simulink library "HDL_ieee_8021513"  (R2024a)
settings: Solver=FixedStepDiscrete  StartTime=0.0  StopTime=10.0  RelTol=1e-3
undefined symbols (not defined in the file): Add, axiWidth, CONST, fs, peakDetectorThreshold, peakDetectorWindow, QAM, Shift
libraries: hdlsllib x199, $bdroot x91, whdlutilities x34, whdledac x9, simulink x8, whdlmod x6, dspsigops x5, dsphdlfiltering2 x4, embreciprocals x3, dsphdlsigops2 x2, commhdlcrc x2, dspstat3 x2
(part 4 of 6)

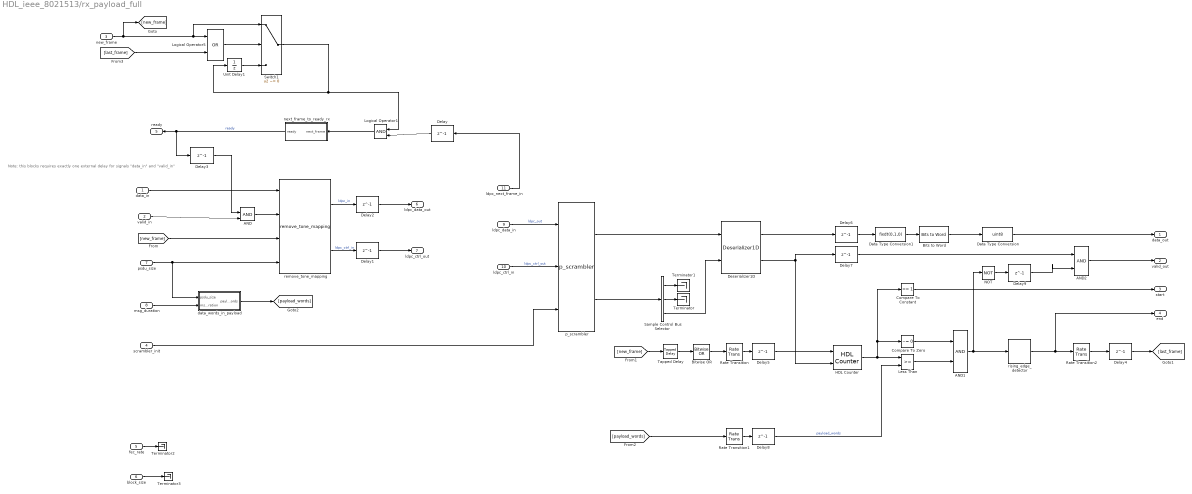
== system HDL_ieee_8021513/rx_payload_full ==
  note: Note: this blocks requires exactly one external delay for signals "data_in" and "valid_in"
  data_in : Inport
  valid_in : Inport  Port=2
  new_frame : Inport  Port=3
  scrambler_init : Inport  Port=4
  fec_rate : Inport  Port=5
  block_size : Inport  Port=6
  psdu_size : Inport  Port=7
  msg_duration : Inport  Port=8
  ldpc_data_in : Inport  Port=9
  ldpc_ctrl_in : Inport  Port=10
  ldpc_next_frame_in : Inport  Port=11
  AND : Logic  IconShape=distinctive  AllPortsSameDT=off  OutDataTypeStr=boolean
  AND1 : Logic  IconShape=distinctive  AllPortsSameDT=off  OutDataTypeStr=boolean
  AND2 : Logic  IconShape=distinctive  AllPortsSameDT=off  OutDataTypeStr=boolean
  Bits to Word : hdlsllib/Logic and Bit Operations/Bits to Word
  Bitwise OR : simulink/Logic and Bit Operations/Bitwise Operator  logicop=OR  UseBitMask=off  BitMask=bin2dec('11011001')  BitMaskRealWorld=Stored Integer
      settings: LibrarySourceBlock=|
      | simulink/Quick Insert/Logic and Bit
      | Operations/Bitwise OR
  Compare To Constant : hdlsllib/Logic and Bit Operations/Compare To Constant  relop===  const=1  OutDataTypeStr=boolean
  Compare To Zero : hdlsllib/Logic and Bit Operations/Compare To Zero  relop=~=  OutDataTypeStr=boolean
  Data Type Conversion : DataTypeConversion  OutDataTypeStr=uint8  SaturateOnIntegerOverflow=off  RndMeth=Floor
  Data Type Conversion1 : DataTypeConversion  OutDataTypeStr=fixdt(0,1,0)  SaturateOnIntegerOverflow=off  RndMeth=Floor
  Delay{,1..9} (10 alike) : Delay  DelayLength=1  InitialCondition=0  UseCircularBuffer=on
  Deserializer1D : hdlsllib/HDL Operations/Deserializer1D  Ratio=8  IdleCycles=0  InitialCondition=0  startIn=off  validIn=on  validOut=on  inputDataDimensions=-1  inputSampleTime=-1  inputSignalType=auto
  HDL Counter : hdlsllib/Sources/HDL Counter  CountType=Free running  CountInit=0  CountStep=1  CountMax=25  CountFromType=Initial value  CountFrom=0  CountResetPort=on  CountLoadPort=off  CountEnbPort=on  CountDirPort=off  CountHitOutputPort=off  CountDataType=Unsigned  CountWordLen=32  CountFracLen=0  CountSampTime=1
  Less Than : RelationalOperator  OutDataTypeStr=boolean  RndMeth=Simplest  InputSameDT=off
  Logical Operator1 : Logic  IconShape=distinctive  AllPortsSameDT=off  OutDataTypeStr=boolean
  Logical Operator5 : Logic  Operator=OR  IconShape=distinctive  AllPortsSameDT=off  OutDataTypeStr=boolean
  NOT : Logic  Operator=NOT  IconShape=distinctive  AllPortsSameDT=off  OutDataTypeStr=boolean
  Rate Transition : RateTransition  OutPortSampleTimeOpt=Multiple of input port sample time  OutPortSampleTimeMultiple=8
  Rate Transition1 : RateTransition  OutPortSampleTimeOpt=Multiple of input port sample time  OutPortSampleTimeMultiple=8
  Rate Transition2 : RateTransition  OutPortSampleTimeOpt=Multiple of input port sample time  OutPortSampleTimeMultiple=1/8
  Sample Control Bus Selector : whdlutilities/Sample Control Bus Selector  OutputSignals=start,end,valid
  Switch1 : Switch  Criteria=u2 ~= 0  SaturateOnIntegerOverflow=off  InputSameDT=off
  Tapped Delay : simulink/Discrete/Tapped Delay  vinit=0.0  samptime=-1  NumDelays=8  DelayOrder=Oldest  includeCurrent=off
  Terminator{,1..3} (4 alike) : Terminator
  Unit Delay1 : UnitDelay  SampleTime=-1  HasFrameUpgradeWarning=on
  data_words_in_payload : Subsystem
  next_frame_to_ready_rx : Subsystem
  p_scrambler : $bdroot/p_scrambler  SystemSampleTime=-1  VariantActivationTime=update diagram  AllowFlexibleInterface=on  Latency=0  AutoFrameSizeCalculation=off
      settings: LibrarySourceBlock=|
      | hdlsllib/Ports &
      | Subsystems/Subsystem
  remove_tone_mapping : $bdroot/remove_tone_mapping  SystemSampleTime=-1  VariantActivationTime=update diagram  AllowFlexibleInterface=on  Latency=0  AutoFrameSizeCalculation=off
  rising_edge_detector : $bdroot/rising_edge_detector  SystemSampleTime=-1  VariantActivationTime=update diagram  AllowFlexibleInterface=on  Latency=0  AutoFrameSizeCalculation=off
  data_out : Outport  VectorParamsAs1DForOutWhenUnconnected=off
  valid_out : Outport  Port=2  VectorParamsAs1DForOutWhenUnconnected=off
  start : Outport  Port=3  VectorParamsAs1DForOutWhenUnconnected=off
  end : Outport  Port=4  VectorParamsAs1DForOutWhenUnconnected=off
  ready : Outport  Port=5  VectorParamsAs1DForOutWhenUnconnected=off
  ldpc_data_out : Outport  Port=6  VectorParamsAs1DForOutWhenUnconnected=off
  ldpc_ctrl_out : Outport  Port=7  VectorParamsAs1DForOutWhenUnconnected=off
  wires:
  Delay6/1 -> Data Type Conversion1/1
  Delay9/1 -> AND2/2
  NOT/1 -> Delay9/1
  AND2/1 -> valid_out/1
  Delay7/1 -> AND2/1
  Compare To Zero/1 -> AND1/1
  Less Than/1 -> AND1/2
  AND1/1 -> rising_edge_detector/1, NOT/1
  Compare To Constant/1 -> start/1
  Delay4/1 -> [last_frame]
  Rate Transition2/1 -> Delay4/1
  rising_edge_detector/1 -> Rate Transition2/1, end/1
  Delay8/1 -> Less Than/2  "payload_words"
  Rate Transition1/1 -> Delay8/1
  [payload_words] -> Rate Transition1/1
  Delay5/1 -> HDL Counter/1
  data_words_in_payload/1(payload_words) -> [payload_words]
  HDL Counter/1 -> Less Than/1, Compare To Zero/1, Compare To Constant/1
  Rate Transition/1 -> Delay5/1
  Bitwise OR/1 -> Rate Transition/1
  [new_frame] -> Tapped Delay/1
  Tapped Delay/1 -> Bitwise OR/1
  msg_duration/1 -> data_words_in_payload/2(msg_duration)
  Deserializer1D/1 -> Delay6/1
  Deserializer1D/2 -> HDL Counter/2, Delay7/1
  Bits to Word/1 -> Data Type Conversion/1
  block_size/1 -> Terminator3/1
  fec_rate/1 -> Terminator2/1
  Delay2/1 -> ldpc_data_out/1
  Delay1/1 -> ldpc_ctrl_out/1
  p_scrambler/2 -> Sample Control Bus Selector/1
  Sample Control Bus Selector/2 -> Terminator/1
  Sample Control Bus Selector/1 -> Terminator1/1
  scrambler_init/1 -> p_scrambler/3
  ldpc_ctrl_in/1 -> p_scrambler/2  "ldpc_ctrl_out"
  ldpc_data_in/1 -> p_scrambler/1  "ldpc_out"
  psdu_size/1 -> remove_tone_mapping/4, data_words_in_payload/1(psdu_size)
  remove_tone_mapping/1 -> Delay2/1  "ldpc_in"
  remove_tone_mapping/2 -> Delay1/1  "ldpc_ctrl_in"
  ldpc_next_frame_in/1 -> Delay/1
  next_frame_to_ready_rx/1(ready) -> Delay3/1, ready/1  "ready"
  data_in/1 -> remove_tone_mapping/1
  AND/1 -> remove_tone_mapping/2
  valid_in/1 -> AND/2
  Delay3/1 -> AND/1
  Logical Operator5/1 -> Switch1/2
  new_frame/1 -> [new_frame], Switch1/1, Logical Operator5/1
  Unit Delay1/1 -> Switch1/3
  Logical Operator1/1 -> next_frame_to_ready_rx/1(next_frame)
  Switch1/1 -> Logical Operator1/1, Unit Delay1/1
  Delay/1 -> Logical Operator1/2
  [last_frame] -> Logical Operator5/2
  [new_frame] -> remove_tone_mapping/3
  Sample Control Bus Selector/3 -> Deserializer1D/2
  Data Type Conversion/1 -> data_out/1
  p_scrambler/1 -> Deserializer1D/1
  Data Type Conversion1/1 -> Bits to Word/1

== system HDL_ieee_8021513/signal_ack ==
  signal_in : Inport
  free_signal : Inport  Port=2
  Logical Operator : Logic  Operator=OR  IconShape=distinctive  AllPortsSameDT=off  OutDataTypeStr=boolean
  Logical Operator3 : Logic  Operator=NOT  IconShape=distinctive  AllPortsSameDT=off  OutDataTypeStr=boolean
  State Control : StateControl  StateControl=Synchronous
  Switch : Switch  Criteria=u2 ~= 0  SaturateOnIntegerOverflow=off  InputSameDT=off
  Unit Delay : UnitDelay  SampleTime=-1  HasFrameUpgradeWarning=on
  rising_edge_detector : $bdroot/rising_edge_detector  SystemSampleTime=-1  VariantActivationTime=update diagram  AllowFlexibleInterface=on  Latency=0  AutoFrameSizeCalculation=off
  signal_out : Outport
  wires:
  Unit Delay/1 -> Switch/3
  Switch/1 -> Logical Operator3/1, Unit Delay/1
  Logical Operator/1 -> Switch/2
  free_signal/1 -> Logical Operator/1, Switch/1
  Logical Operator3/1 -> signal_out/1
  signal_in/1 -> rising_edge_detector/1
  rising_edge_detector/1 -> Logical Operator/2

== system HDL_ieee_8021513/tone_mapping ==
  data_in : Inport
  ctrl_in : Inport  Port=2
  bits_per_subcarrier : Inport  Port=3
  len_in_ofdm_symbols : Inport  Port=4
  new_frame : Inport  Port=5
  Compare To Constant : hdlsllib/Logic and Bit Operations/Compare To Constant  relop===  const=1  OutDataTypeStr=boolean
  Constant : Constant  Value=0  OutDataTypeStr=boolean  SampleTime=-1
  Data Type Conversion : DataTypeConversion  OutDataTypeStr=uint8  SaturateOnIntegerOverflow=off  RndMeth=Floor
  Delay{,1..4,6..7,10} (8 alike) : Delay  DelayLength=1  InitialCondition=0  UseCircularBuffer=on
  Delay{5,8..9,11..12} (5 alike) : Delay  InitialCondition=0  UseCircularBuffer=on
  Gain : Gain  Gain=CONST.numDataCarriers  OutDataTypeStr=fixdt(0,10,0)
  HDL Counter : hdlsllib/Sources/HDL Counter  CountType=Free running  CountInit=0  CountStep=1  CountMax=1  CountFromType=Initial value  CountFrom=0  CountResetPort=on  CountLoadPort=off  CountEnbPort=on  CountDirPort=off  CountHitOutputPort=off  CountDataType=Unsigned  CountWordLen=32  CountFracLen=0  CountSampTime=1
  Logical Operator : Logic  AllPortsSameDT=off  OutDataTypeStr=boolean
  Logical Operator1 : Logic  IconShape=distinctive  AllPortsSameDT=off  OutDataTypeStr=boolean
  Logical Operator{2,4,6..7} (4 alike) : Logic  Operator=OR  IconShape=distinctive  AllPortsSameDT=off  OutDataTypeStr=boolean
  Logical Operator3 : Logic  IconShape=distinctive  AllPortsSameDT=off  OutDataTypeStr=boolean
  Logical Operator5 : Logic  IconShape=distinctive  AllPortsSameDT=off  OutDataTypeStr=boolean
  Product1 : Product
  Relational Operator : RelationalOperator  Operator=<=  OutDataTypeStr=boolean  InputSameDT=off
  Sample Control Bus Creator : whdlutilities/Sample Control Bus Creator
  Sample Control Bus Selector : whdlutilities/Sample Control Bus Selector  OutputSignals=start,end,valid
  State Control : StateControl  StateControl=Synchronous
  Subtract : Sum  Inputs=+-
  Switch : Switch  Criteria=u2 ~= 0  SaturateOnIntegerOverflow=off  InputSameDT=off
  Switch1 : Switch  Criteria=u2 ~= 0  SaturateOnIntegerOverflow=off  InputSameDT=off
  Switch2 : Switch  Criteria=u2 ~= 0  SaturateOnIntegerOverflow=off  InputSameDT=off
  Unit Delay1 : UnitDelay  SampleTime=-1  HasFrameUpgradeWarning=on
  Unit Delay2 : UnitDelay  SampleTime=-1  HasFrameUpgradeWarning=on
  data_out : Outport
  ctrl_out : Outport  Port=2
  wires:
  Delay12/1 -> Delay9/1
  Delay11/1 -> Gain/1
  Data Type Conversion/1 -> Delay11/1
  Delay2/1 -> Logical Operator7/1
  Logical Operator1/1 -> Delay3/1
  Logical Operator7/1 -> Switch1/2
  Sample Control Bus Selector/1 -> Logical Operator1/2, Delay2/1
  Unit Delay2/1 -> Switch1/3
  Switch1/1 -> Unit Delay2/1, Logical Operator1/1  "new_frame_hold"
  Sample Control Bus Selector/2 -> Logical Operator/1
  Relational Operator/1 -> Logical Operator/2
  Logical Operator/1 -> Switch2/1, Logical Operator6/2
  new_frame/1 -> Logical Operator7/2, Switch1/1, HDL Counter/1  "new_frame"
  Switch/1 -> data_out/1
  ctrl_in/1 -> Delay7/1
  Sample Control Bus Selector/3 -> Delay10/1
  Sample Control Bus Creator/1 -> ctrl_out/1
  Logical Operator2/1 -> Sample Control Bus Creator/3
  Unit Delay1/1 -> Switch2/3
  Switch2/1 -> Delay1/1, Unit Delay1/1
  Logical Operator3/1 -> Sample Control Bus Creator/2
  Logical Operator4/1 -> HDL Counter/2  "enable"
  [hold_end] -> Logical Operator4/2
  Constant/1 -> Switch/1
  data_in/1 -> Delay6/1
  [hold_end] -> Logical Operator3/2
  HDL Counter/1 -> Subtract/2  "count"
  Delay/1 -> Switch/3
  Delay1/1 -> [hold_end], Logical Operator5/2, Logical Operator2/2  "hold_end"
  Delay10/1 -> Logical Operator4/1, Logical Operator2/1
  Delay3/1 -> Sample Control Bus Creator/1
  Logical Operator6/1 -> Switch2/2
  Logical Operator5/1 -> Logical Operator6/1
  [hold_end] -> Delay4/1
  Delay4/1 -> Switch/2
  Subtract/1 -> Relational Operator/1, Compare To Constant/1
  Compare To Constant/1 -> Logical Operator5/1, Logical Operator3/1
  bits_per_subcarrier/1 -> Data Type Conversion/1
  Delay5/1 -> [count_hit]  "count_hit"
  [count_hit] -> Subtract/1
  Delay6/1 -> Delay/1
  Delay7/1 -> Sample Control Bus Selector/1
  Gain/1 -> Delay8/1
  Delay8/1 -> Product1/1, Relational Operator/2
  len_in_ofdm_symbols/1 -> Delay12/1
  Product1/1 -> Delay5/1
  Delay9/1 -> Product1/2

== system HDL_ieee_8021513/tx_decimator ==
  note: The data out from this blocks is "valid" one sample, and invalid the next.
      | This blocks makes sure that the data is valid both cycles.
      | What happens is that the ZOH might sample the signal when is valid or invalid.
  data_in : Inport
  valid_in : Inport  Port=2
  Delay{,1..2,5..10} (9 alike) : Delay  DelayLength=1  InitialCondition=0  UseCircularBuffer=on
  Delay3 : Delay  DelayLength=CONST.txDecimatorDelay*3 +6  InitialCondition=0  UseCircularBuffer=on
  Delay4 : Delay  DelayLength=CONST.txDecimatorDelay/CONST.txM  InitialCondition=0  UseCircularBuffer=on
  Downsample : DownSample  N=CONST.txM  RateOptions=Allow multirate processing
  Downsample1 : DownSample  N=CONST.txM  RateOptions=Allow multirate processing
  FIR Decimator : dsphdlfiltering2/FIR Decimator  Numerator=CONST.txDecimatorFilter.Numerator  FilterStructure=Direct form systolic  DecimationFactor=CONST.txM  NumCycles=1  SimulateUsing=Code generation  roundingMode=Floor  overflowMode=off  CoefficientsDataTypeStr=fixdt(1,16)  OutputDataTypeStr=fixdt(1,16,12)  ResetInputPort=on  HDLGlobalReset=on
  Logical Operator : Logic  Operator=OR  IconShape=distinctive  AllPortsSameDT=off  OutDataTypeStr=boolean
  Logical Operator2 : Logic  IconShape=distinctive  AllPortsSameDT=off  OutDataTypeStr=boolean
  Logical Operator3 : Logic  IconShape=distinctive  AllPortsSameDT=off  OutDataTypeStr=boolean
  Logical Operator4 : Logic  Operator=NOT  IconShape=distinctive  AllPortsSameDT=off  OutDataTypeStr=boolean
  Switch : Switch  Criteria=u2 ~= 0  SaturateOnIntegerOverflow=off  InputSameDT=off
  Switch1 : Switch  Criteria=u2 ~= 0  SaturateOnIntegerOverflow=off  InputSameDT=off
  falling_edge_detector : $bdroot/falling_edge_detector  SystemSampleTime=-1  VariantActivationTime=update diagram  AllowFlexibleInterface=on  Latency=0  AutoFrameSizeCalculation=off
  rising_edge_detector : $bdroot/rising_edge_detector  SystemSampleTime=-1  VariantActivationTime=update diagram  AllowFlexibleInterface=on  Latency=0  AutoFrameSizeCalculation=off
  data_out : Outport
  valid_out : Outport  Port=2
  wires:
  rising_edge_detector/1 -> FIR Decimator/3
  Delay10/1 -> Delay5/1
  Delay1/1 -> Logical Operator/1, Delay3/1
  valid_in/1 -> Delay1/1, rising_edge_detector/1
  Downsample1/1 -> Delay2/1
  Delay3/1 -> Logical Operator/2
  Logical Operator/1 -> FIR Decimator/2
  data_in/1 -> Delay10/1  "data_in"
  Downsample/1 -> Delay8/1  "after_down"
  Delay5/1 -> FIR Decimator/1
  Delay6/1 -> Switch/3
  Delay7/1 -> Switch1/3
  Switch1/1 -> Downsample/1
  FIR Decimator/1 -> Switch/1, Delay6/1  "data_out"
  Switch/1 -> Downsample1/1
  FIR Decimator/2 -> Delay7/1, Switch/2, Switch1/1, Switch1/2  "valid_out"
  Delay/1 -> Logical Operator3/1
  Logical Operator4/1 -> Logical Operator3/2
  Delay9/1 -> data_out/1
  Logical Operator2/1 -> Delay/1, falling_edge_detector/1
  Delay8/1 -> Logical Operator2/1, Delay4/1
  Logical Operator3/1 -> valid_out/1
  falling_edge_detector/1 -> Logical Operator4/1
  Delay4/1 -> Logical Operator2/2
  Delay2/1 -> Delay9/1

== system HDL_ieee_8021513/valid_to_ctrl ==
  validIn : Inport
  Delay1 : Delay  DelayLength=1  InitialCondition=0  UseCircularBuffer=on
  Delay2 : Delay  DelayLength=1  InitialCondition=0  UseCircularBuffer=on
  Logical Operator : Logic  IconShape=distinctive  AllPortsSameDT=off  OutDataTypeStr=boolean
  Logical Operator1 : Logic  Operator=NOT  IconShape=distinctive  AllPortsSameDT=off  OutDataTypeStr=boolean
  Logical Operator2 : Logic  IconShape=distinctive  AllPortsSameDT=off  OutDataTypeStr=boolean
  Logical Operator3 : Logic  Operator=NOT  IconShape=distinctive  AllPortsSameDT=off  OutDataTypeStr=boolean
  Sample Control Bus Creator : whdlutilities/Sample Control Bus Creator
  State Control : StateControl  StateControl=Synchronous
  ctrlOut : Outport  VectorParamsAs1DForOutWhenUnconnected=off
  wires:
  validIn/1 -> Logical Operator3/1, Delay1/1
  Logical Operator3/1 -> Logical Operator2/2
  Delay2/1 -> Logical Operator1/1
  Logical Operator1/1 -> Logical Operator/2
  Delay1/1 -> Logical Operator/1, Sample Control Bus Creator/3, Logical Operator2/1, Delay2/1  "valid"
  Logical Operator/1 -> Sample Control Bus Creator/1  "start"
  Logical Operator2/1 -> Sample Control Bus Creator/2  "end"
  Sample Control Bus Creator/1 -> ctrlOut/1

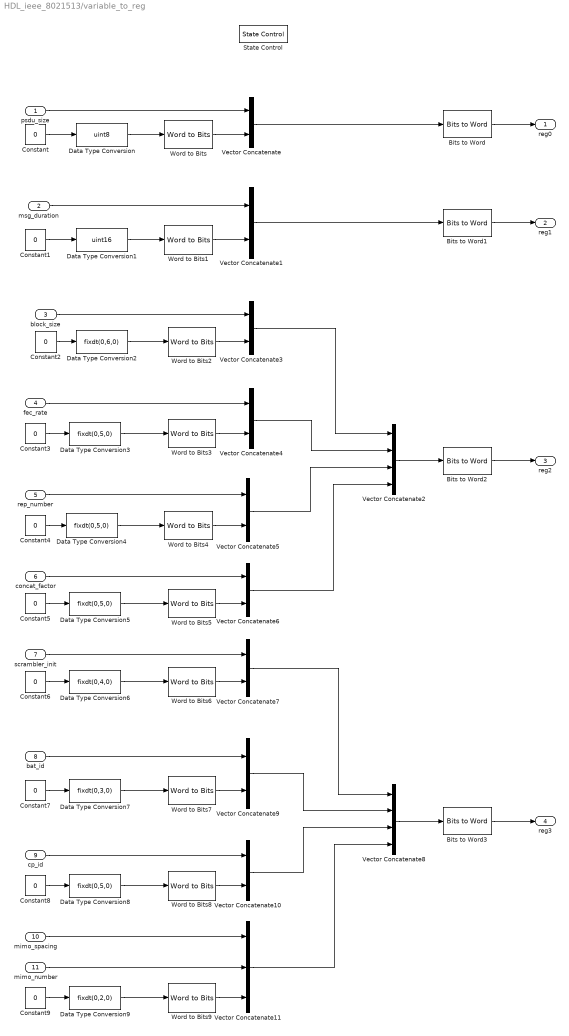
== system HDL_ieee_8021513/variable_to_reg ==
  psdu_size : Inport
  msg_duration : Inport  Port=2
  block_size : Inport  Port=3
  fec_rate : Inport  Port=4
  rep_number : Inport  Port=5
  concat_factor : Inport  Port=6
  scrambler_init : Inport  Port=7
  bat_id : Inport  Port=8
  cp_id : Inport  Port=9
  mimo_spacing : Inport  Port=10
  mimo_number : Inport  Port=11
  Bits to Word{,1..3} (4 alike) : hdlsllib/Logic and Bit Operations/Bits to Word
  Constant : Constant  Value=0  OutDataTypeStr=uint8  SampleTime=-1
  Constant1 : Constant  Value=0  OutDataTypeStr=uint16  SampleTime=-1
  Constant2 : Constant  Value=0  OutDataTypeStr=fixdt(0,6,0)  SampleTime=-1
  Constant{3..5,8} (4 alike) : Constant  Value=0  OutDataTypeStr=fixdt(0,5,0)  SampleTime=-1
  Constant6 : Constant  Value=0  OutDataTypeStr=fixdt(0,4,0)  SampleTime=-1
  Constant7 : Constant  Value=0  OutDataTypeStr=fixdt(0,3,0)  SampleTime=-1
  Constant9 : Constant  Value=0  OutDataTypeStr=fixdt(0,2,0)  SampleTime=-1
  Data Type Conversion : DataTypeConversion  OutDataTypeStr=uint8  SaturateOnIntegerOverflow=off  RndMeth=Floor
  Data Type Conversion1 : DataTypeConversion  OutDataTypeStr=uint16  SaturateOnIntegerOverflow=off  RndMeth=Floor
  Data Type Conversion2 : DataTypeConversion  OutDataTypeStr=fixdt(0,6,0)  SaturateOnIntegerOverflow=off  RndMeth=Floor
  Data Type Conversion{3..5,8} (4 alike) : DataTypeConversion  OutDataTypeStr=fixdt(0,5,0)  SaturateOnIntegerOverflow=off  RndMeth=Floor
  Data Type Conversion6 : DataTypeConversion  OutDataTypeStr=fixdt(0,4,0)  SaturateOnIntegerOverflow=off  RndMeth=Floor
  Data Type Conversion7 : DataTypeConversion  OutDataTypeStr=fixdt(0,3,0)  SaturateOnIntegerOverflow=off  RndMeth=Floor
  Data Type Conversion9 : DataTypeConversion  OutDataTypeStr=fixdt(0,2,0)  SaturateOnIntegerOverflow=off  RndMeth=Floor
  State Control : StateControl  StateControl=Synchronous
  Vector Concatenate{,1,3..7,9..10} (9 alike) : Concatenate
  Vector Concatenate11 : Concatenate  NumInputs=3
  Vector Concatenate2 : Concatenate  NumInputs=4
  Vector Concatenate8 : Concatenate  NumInputs=4
  Word to Bits : hdlsllib/Logic and Bit Operations/Word to Bits  maxWordLength=8
  Word to Bits1 : hdlsllib/Logic and Bit Operations/Word to Bits  maxWordLength=16
  Word to Bits2 : hdlsllib/Logic and Bit Operations/Word to Bits  maxWordLength=6
  Word to Bits{3..5,8} (4 alike) : hdlsllib/Logic and Bit Operations/Word to Bits  maxWordLength=5
  Word to Bits6 : hdlsllib/Logic and Bit Operations/Word to Bits  maxWordLength=4
  Word to Bits7 : hdlsllib/Logic and Bit Operations/Word to Bits  maxWordLength=3
  Word to Bits9 : hdlsllib/Logic and Bit Operations/Word to Bits  maxWordLength=2
  reg0 : Outport
  reg1 : Outport  Port=2
  reg2 : Outport  Port=3
  reg3 : Outport  Port=4
  wires:
  psdu_size/1 -> Vector Concatenate/1
  Constant/1 -> Data Type Conversion/1
  Word to Bits/1 -> Vector Concatenate/2
  Vector Concatenate/1 -> Bits to Word/1
  Bits to Word/1 -> reg0/1
  Data Type Conversion/1 -> Word to Bits/1
  Constant1/1 -> Data Type Conversion1/1
  Data Type Conversion1/1 -> Word to Bits1/1
  msg_duration/1 -> Vector Concatenate1/1
  Word to Bits1/1 -> Vector Concatenate1/2
  Vector Concatenate1/1 -> Bits to Word1/1
  Bits to Word1/1 -> reg1/1
  Constant2/1 -> Data Type Conversion2/1
  Data Type Conversion2/1 -> Word to Bits2/1
  block_size/1 -> Vector Concatenate3/1
  Word to Bits2/1 -> Vector Concatenate3/2
  Constant3/1 -> Data Type Conversion3/1
  Data Type Conversion3/1 -> Word to Bits3/1
  fec_rate/1 -> Vector Concatenate4/1
  Word to Bits3/1 -> Vector Concatenate4/2
  Vector Concatenate3/1 -> Vector Concatenate2/1
  Vector Concatenate4/1 -> Vector Concatenate2/2
  Vector Concatenate2/1 -> Bits to Word2/1
  Constant4/1 -> Data Type Conversion4/1
  Data Type Conversion4/1 -> Word to Bits4/1
  rep_number/1 -> Vector Concatenate5/1
  Word to Bits4/1 -> Vector Concatenate5/2
  Vector Concatenate5/1 -> Vector Concatenate2/3
  Data Type Conversion5/1 -> Word to Bits5/1
  Constant5/1 -> Data Type Conversion5/1
  concat_factor/1 -> Vector Concatenate6/1
  Word to Bits5/1 -> Vector Concatenate6/2
  Vector Concatenate6/1 -> Vector Concatenate2/4
  Data Type Conversion6/1 -> Word to Bits6/1
  Constant6/1 -> Data Type Conversion6/1
  scrambler_init/1 -> Vector Concatenate7/1
  Word to Bits6/1 -> Vector Concatenate7/2
  Vector Concatenate7/1 -> Vector Concatenate8/1
  Constant7/1 -> Data Type Conversion7/1
  Data Type Conversion7/1 -> Word to Bits7/1
  bat_id/1 -> Vector Concatenate9/1
  Word to Bits7/1 -> Vector Concatenate9/2
  Vector Concatenate9/1 -> Vector Concatenate8/2
  Data Type Conversion8/1 -> Word to Bits8/1
  Constant8/1 -> Data Type Conversion8/1
  cp_id/1 -> Vector Concatenate10/1
  Word to Bits8/1 -> Vector Concatenate10/2
  mimo_spacing/1 -> Vector Concatenate11/1
  mimo_number/1 -> Vector Concatenate11/2
  Constant9/1 -> Data Type Conversion9/1
  Data Type Conversion9/1 -> Word to Bits9/1
  Word to Bits9/1 -> Vector Concatenate11/3
  Vector Concatenate10/1 -> Vector Concatenate8/3
  Vector Concatenate11/1 -> Vector Concatenate8/4
  Vector Concatenate8/1 -> Bits to Word3/1
  Bits to Word2/1 -> reg2/1
  Bits to Word3/1 -> reg3/1

== system HDL_ieee_8021513/calculate_mean_and_std/calculate_mean_x ==
  note: Return:
      | $\sum_{i=0}^{N-1}{x(i)}$
  data_in : Inport
  Add1 : Sum  OutDataTypeStr=Inherit: Same as first input
  Delay : Delay  DelayLength=1  InitialCondition=0  UseCircularBuffer=on
  Delay1 : Delay  DelayLength=1  InitialCondition=0  UseCircularBuffer=on
  Delay2 : Delay  DelayLength=1  InitialCondition=0  UseCircularBuffer=on
  Divide by 1024 : hdlsllib/Logic and Bit Operations/Bit Shift  mode=Shift Right Arithmetic  N=10
  N delay : Delay  DelayLength=1024  InitialCondition=0  UseCircularBuffer=on
  Subtract : Sum  Inputs=+-  OutDataTypeStr=fixdt(1,32,12)
  mean : Outport
  wires:
  data_in/1 -> Delay2/1  "x(i+N)"
  Delay1/1 -> Divide by 1024/1, Add1/2
  N delay/1 -> Subtract/2  "x(i)"
  Add1/1 -> Delay1/1
  Subtract/1 -> Delay/1
  Divide by 1024/1 -> mean/1
  Delay/1 -> Add1/1
  Delay2/1 -> Subtract/1, N delay/1

== system HDL_ieee_8021513/calculate_mean_and_std/calculate_mean_x_squared ==
  note: Return:
      | $\sum_{i=0}^{N-1}{(x(i)^2)}$
  data_in : Inport
  Add1 : Sum  OutDataTypeStr=Inherit: Same as first input
  Delay : Delay  DelayLength=1  InitialCondition=0  UseCircularBuffer=on
  Delay1 : Delay  DelayLength=1  InitialCondition=0  UseCircularBuffer=on
  Delay2 : Delay  DelayLength=1  InitialCondition=0  UseCircularBuffer=on
  Divide by 1024 : hdlsllib/Logic and Bit Operations/Bit Shift  mode=Shift Right Arithmetic  N=10
  N delay : Delay  DelayLength=1024  InitialCondition=0  UseCircularBuffer=on
  Square : Math  Operator=square  SignedPower=on  RndMeth=Zero  OutDataTypeStr=Inherit: Inherit via internal rule
  Subtract : Sum  Inputs=+-
  mean_x_squared : Outport
  wires:
  data_in/1 -> Square/1  "x(i+N)"
  Delay1/1 -> Divide by 1024/1, Add1/2
  N delay/1 -> Subtract/2  "x(i)"
  Add1/1 -> Delay1/1
  Subtract/1 -> Delay/1
  Divide by 1024/1 -> mean_x_squared/1
  Delay/1 -> Add1/1
  Square/1 -> Delay2/1
  Delay2/1 -> Subtract/1, N delay/1

== system HDL_ieee_8021513/channel_estimation_and_equalization/Channel Equalization ==
  note: Latency divider:
      | 10 + nextpow2(u.WordLength) + u.WordLength
  data_in : Inport
  valid_data : Inport  Port=2
  channel_estimate_in : Inport  Port=3
  valid_channel_estimate : Inport  Port=4
  Channel Estimates Store RAM : hdlsllib/HDL RAMs/Simple Dual Port RAM System  RAMType=Simple dual port  AsyncRead=off  WriteOutputValue=New data  RAMInitialValue=0  allowBusInputs=off  WritesHaveOutput=on  NumReads=0  NumWrites=1  SimulateUsing=Code generation
  Delay : Delay  DelayLength=1
  Delay1 : Delay  DelayLength=6  InitialCondition=0  UseCircularBuffer=on
  Delay12 : Delay  DelayLength=CONST.rxChannelEstDividerDelay  InitialCondition=0  UseCircularBuffer=on
  Delay23 : Delay  DelayLength=1  InitialCondition=0
  Delay24 : Delay  DelayLength=1  InitialCondition=0
  Delay25 : Delay  DelayLength=1  InitialCondition=0
  Delay28 : Delay  DelayLength=1
  Delay{3..6} (4 alike) : Delay  DelayLength=1  InitialCondition=0  UseCircularBuffer=on
  HDL Counter : hdlsllib/Sources/HDL Counter  CountType=Count limited  CountInit=0  CountStep=1  CountMax=CONST.numDataCarriers-1  CountFromType=Initial value  CountFrom=0  CountResetPort=on  CountLoadPort=off  CountEnbPort=on  CountDirPort=off  CountHitOutputPort=off  CountDataType=Unsigned  CountWordLen=nextpow2(CONST.numDataCarriers)  CountFracLen=0  CountSampTime=1
  HDL Counter1 : hdlsllib/Sources/HDL Counter  CountType=Count limited  CountInit=0  CountStep=1  CountMax=CONST.numDataCarriers-1  CountFromType=Initial value  CountFrom=0  CountResetPort=on  CountLoadPort=off  CountEnbPort=on  CountDirPort=off  CountHitOutputPort=off  CountDataType=Unsigned  CountWordLen=nextpow2(CONST.numDataCarriers)  CountFracLen=0  CountSampTime=1
  equalizer : Subsystem
  rising_edge_detector : $bdroot/rising_edge_detector  SystemSampleTime=-1  VariantActivationTime=update diagram  AllowFlexibleInterface=on  Latency=0  AutoFrameSizeCalculation=off
  rising_edge_detector1 : $bdroot/rising_edge_detector  SystemSampleTime=-1  VariantActivationTime=update diagram  AllowFlexibleInterface=on  Latency=0  AutoFrameSizeCalculation=off
  data_out : Outport
  valid_out : Outport  Port=2
  channel_est_out : Outport  Port=3
  wires:
  equalizer/2(valid_out) -> valid_out/1
  equalizer/1(data_out) -> data_out/1
  Delay25/1 -> equalizer/3(Valid)  "Valid"
  Delay24/1 -> equalizer/1(data_in)
  Delay1/1 -> Delay12/1
  Delay12/1 -> channel_est_out/1
  Delay6/1 -> Delay/1
  Delay5/1 -> Channel Estimates Store RAM/1
  Delay4/1 -> HDL Counter1/2, Delay28/1
  Delay3/1 -> HDL Counter/2, Channel Estimates Store RAM/3
  rising_edge_detector1/1 -> HDL Counter/1
  rising_edge_detector/1 -> HDL Counter1/1
  Channel Estimates Store RAM/1 -> Delay23/1
  HDL Counter1/1 -> Channel Estimates Store RAM/4  "rdAddr"
  valid_data/1 -> Delay4/1, rising_edge_detector/1
  valid_channel_estimate/1 -> Delay3/1, rising_edge_detector1/1
  HDL Counter/1 -> Channel Estimates Store RAM/2
  Delay/1 -> Delay24/1
  Delay28/1 -> Delay25/1
  data_in/1 -> Delay6/1
  channel_estimate_in/1 -> Delay5/1
  Delay23/1 -> equalizer/2(hEst), Delay1/1  "hEst"

== system HDL_ieee_8021513/channel_estimation_and_equalization/Channel Estimation ==
  note: Modificacion del channel estimation, para reducir DSPs, considerando que el valor de referencia del canal es H="-1 + 0i"
  note: Store first channel symbol
  data_in : Inport
  valid_in : Inport  Port=2
  reset : Inport  Port=3
  Add : Sum
  Data Type Conversion : DataTypeConversion  OutDataTypeStr=fixdt(1, CONST.rxChannelEstReferenceWordLength, CONST.rxChannelEstReferenceFractionLength)  SaturateOnIntegerOverflow=off  RndMeth=Floor
  Delay{,1..8} (9 alike) : Delay  DelayLength=1  InitialCondition=0  UseCircularBuffer=on
  Divide by 2 : hdlsllib/Logic and Bit Operations/Bit Shift  mode=Shift Right Arithmetic  N=1
  HDL Counter : hdlsllib/Sources/HDL Counter  CountType=Count limited  CountInit=0  CountStep=1  CountMax=2  CountFromType=Initial value  CountFrom=0  CountResetPort=on  CountLoadPort=off  CountEnbPort=on  CountDirPort=off  CountHitOutputPort=on  CountDataType=Unsigned  CountWordLen=2  CountFracLen=0  CountSampTime=1
  HDL FIFO : hdlsllib/HDL RAMs/HDL FIFO  fifo_size=CONST.numDataCarriers  mode=Classic  ratio=1  push_msg=Error  pop_msg=Error  show_empty=off  show_full=off  show_num=off  LabelModeActiveChoice_Mode=Classic  rst_port=on
  Logical Operator : Logic  Operator=NOT  IconShape=distinctive  AllPortsSameDT=off  OutDataTypeStr=boolean
  Logical Operator1 : Logic  AllPortsSameDT=off  OutDataTypeStr=boolean
  Logical Operator2 : Logic  AllPortsSameDT=off  OutDataTypeStr=boolean
  Terminator : Terminator
  Unary Minus : UnaryMinus
  rising_edge_detector : $bdroot/rising_edge_detector  SystemSampleTime=-1  VariantActivationTime=update diagram  AllowFlexibleInterface=on  Latency=0  AutoFrameSizeCalculation=off
  channel_estimate : Outport
  valid_estimate : Outport  Port=2
  wires:
  Delay8/1 -> Delay2/1, HDL FIFO/1
  Delay7/1 -> Logical Operator2/1
  Delay6/1 -> Logical Operator1/1
  Delay2/1 -> Add/1
  Delay1/1 -> Delay4/1
  HDL FIFO/1 -> Add/2
  [isSecondSymbol] -> Logical Operator2/2
  Logical Operator2/1 -> HDL FIFO/3, Delay1/1
  [isFirstSymbol] -> Logical Operator1/2
  Logical Operator1/1 -> HDL FIFO/2
  valid_in/1 -> Delay6/1, Delay7/1, rising_edge_detector/1
  rising_edge_detector/1 -> HDL Counter/2
  HDL Counter/1 -> Terminator/1
  HDL Counter/2 -> [isSecondSymbol], Logical Operator/1
  Logical Operator/1 -> [isFirstSymbol]
  Unary Minus/1 -> Delay/1
  Data Type Conversion/1 -> Unary Minus/1
  Delay3/1 -> Divide by 2/1
  Add/1 -> Delay3/1
  Delay5/1 -> valid_estimate/1
  Delay/1 -> channel_estimate/1
  reset/1 -> HDL FIFO/4, HDL Counter/1
  data_in/1 -> Delay8/1
  Delay4/1 -> Delay5/1
  Divide by 2/1 -> Data Type Conversion/1

== system HDL_ieee_8021513/constellation_descrambler/rotate_-90 ==
  data_in : Inport
  valid_in : Inport  Port=2
  s1_in : Inport  Port=3
  s2_in : Inport  Port=4
  Delay : Delay  InitialCondition=0  UseCircularBuffer=on
  Delay1 : Delay  InitialCondition=0  UseCircularBuffer=on
  Delay2 : Delay  DelayLength=1  InitialCondition=0  UseCircularBuffer=on
  Delay3 : Delay  DelayLength=1  InitialCondition=0  UseCircularBuffer=on
  rotate_-90 : Subsystem
  data_out : Outport  VectorParamsAs1DForOutWhenUnconnected=off
  valid_out : Outport  Port=2  VectorParamsAs1DForOutWhenUnconnected=off
  wires:
  s2_in/1 -> rotate_-90/1(s2)  "s2"
  s1_in/1 -> rotate_-90/2(s1)  "s1"
  Delay3/1 -> valid_out/1
  Delay2/1 -> data_out/1  "data_out"
  Delay1/1 -> Delay3/1
  rotate_-90/1(data_out) -> Delay2/1  "data_out"
  Delay/1 -> rotate_-90/3(data_in)  "data_in"
  data_in/1 -> Delay/1
  valid_in/1 -> Delay1/1  "en"

== system HDL_ieee_8021513/constellation_scrambler/rotate ==
  data_in : Inport
  valid_in : Inport  Port=2
  s1 : Inport  Port=3
  s2 : Inport  Port=4
  Bit Concat : hdlsllib/Logic and Bit Operations/Bit Concat  numInputs=2
  Complex to Real-Imag : ComplexToRealImag
  Complex to Real-Imag1 : ComplexToRealImag
  Complex to Real-Imag2 : ComplexToRealImag
  Delay : Delay  DelayLength=1  InitialCondition=0  UseCircularBuffer=on
  Delay1 : Delay  DelayLength=1  InitialCondition=0  UseCircularBuffer=on
  Multiport Switch : MultiPortSwitch  DataPortOrder=Zero-based contiguous  Inputs=4  zeroidx=on  SaturateOnIntegerOverflow=off  InputSameDT=off
  Real-Imag to Complex : RealImagToComplex
  Real-Imag to Complex1 : RealImagToComplex
  Real-Imag to Complex2 : RealImagToComplex
  State Control : StateControl  StateControl=Synchronous
  Unary Minus{,1..3} (4 alike) : UnaryMinus
  data_out : Outport
  valid_out : Outport  Port=2
  wires:
  Delay1/1 -> valid_out/1
  Delay/1 -> data_out/1
  valid_in/1 -> Delay1/1
  s2/1 -> Bit Concat/1
  s1/1 -> Bit Concat/2
  Bit Concat/1 -> Multiport Switch/1
  data_in/1 -> Complex to Real-Imag1/1, Complex to Real-Imag2/1, Complex to Real-Imag/1, Multiport Switch/2
  Complex to Real-Imag/1 -> Unary Minus/1
  Unary Minus/1 -> Real-Imag to Complex/1
  Complex to Real-Imag/2 -> Unary Minus3/1
  Real-Imag to Complex/1 -> Multiport Switch/4
  Complex to Real-Imag1/1 -> Real-Imag to Complex1/2
  Complex to Real-Imag1/2 -> Unary Minus1/1
  Unary Minus1/1 -> Real-Imag to Complex1/1
  Real-Imag to Complex1/1 -> Multiport Switch/3
  Complex to Real-Imag2/1 -> Unary Minus2/1
  Unary Minus2/1 -> Real-Imag to Complex2/2
  Complex to Real-Imag2/2 -> Real-Imag to Complex2/1
  Real-Imag to Complex2/1 -> Multiport Switch/5
  Multiport Switch/1 -> Delay/1
  Unary Minus3/1 -> Real-Imag to Complex/2

== system HDL_ieee_8021513/downshifter/digital_carrier_receiver ==
  dataIn : Inport
  ncoIn : Inport  Port=2
  Complex to Real-Imag : ComplexToRealImag
  Delay{,1..5} (6 alike) : Delay  InitialCondition=0  UseCircularBuffer=on
  Product : Product  OutDataTypeStr=Inherit: Same as first input
  Product2 : Product  OutDataTypeStr=Inherit: Same as first input
  Real-Imag to Complex : RealImagToComplex
  Unary Minus : UnaryMinus
  data_out : Outport  VectorParamsAs1DForOutWhenUnconnected=off
  wires:
  Delay2/1 -> Product/1
  Delay1/1 -> Product/2
  Delay3/1 -> Product2/2
  Delay5/1 -> Product2/1
  Complex to Real-Imag/2 -> Delay5/1
  Complex to Real-Imag/1 -> Delay2/1
  ncoIn/1 -> Complex to Real-Imag/1
  Real-Imag to Complex/1 -> data_out/1
  Delay/1 -> Real-Imag to Complex/1
  Delay4/1 -> Real-Imag to Complex/2
  Product/1 -> Delay/1
  Product2/1 -> Delay4/1
  Unary Minus/1 -> Delay3/1
  dataIn/1 -> Delay1/1, Unary Minus/1

== system HDL_ieee_8021513/frequency_upshift/Mixer ==
  dataIn : Inport
  ncoIn : Inport  Port=2
  Add : Sum  Inputs=+-  InputSameDT=on  OutDataTypeStr=Inherit: Same as first input
  Complex to Real-Imag : ComplexToRealImag
  Complex to Real-Imag1 : ComplexToRealImag
  Delay{,5,8..9} (4 alike) : Delay  InitialCondition=0  UseCircularBuffer=on
  Delay{1..4,6..7} (6 alike) : Delay  DelayLength=3  InitialCondition=0
  Delay12 : Delay  InitialCondition=0
  Multiply by two : hdlsllib/Logic and Bit Operations/Bit Shift  mode=Shift Left Logical  N=1
  Product1 : Product  OutDataTypeStr=Inherit: Same as first input
  Product2 : Product  OutDataTypeStr=Inherit: Same as first input
  State Control : StateControl  StateControl=Synchronous
  mixedOut : Outport
  wires:
  Multiply by two/1 -> Delay/1
  Delay8/1 -> Multiply by two/1
  Delay9/1 -> Delay5/1
  Delay5/1 -> Complex to Real-Imag/1
  Delay/1 -> Complex to Real-Imag1/1
  Delay1/1 -> Product1/1
  ncoIn/1 -> Delay8/1
  Product1/1 -> Delay6/1
  Product2/1 -> Delay7/1
  Delay7/1 -> Add/2
  Complex to Real-Imag1/2 -> Delay4/1
  Complex to Real-Imag/1 -> Delay1/1
  Delay6/1 -> Add/1
  Add/1 -> Delay12/1
  Delay4/1 -> Product2/2
  Delay2/1 -> Product2/1
  Delay12/1 -> mixedOut/1
  dataIn/1 -> Delay9/1
  Complex to Real-Imag1/1 -> Delay3/1
  Delay3/1 -> Product1/2
  Complex to Real-Imag/2 -> Delay2/1

== system HDL_ieee_8021513/full_ofdm_modulator/ofdm_ready_truncate ==
  next_frame : Inport
  new_psdu : Inport  Port=2
  Delay : Delay  DelayLength=1  InitialCondition=0  UseCircularBuffer=on
  HDL Counter : hdlsllib/Sources/HDL Counter  CountType=Count limited  CountInit=0  CountStep=1  CountMax=CONST.numDataCarriers-1  CountFromType=Initial value  CountFrom=0  CountResetPort=off  CountLoadPort=off  CountEnbPort=on  CountDirPort=off  CountHitOutputPort=on  CountDataType=Unsigned  CountWordLen=nextpow2(CONST.numDataCarriers)  CountFracLen=0  CountSampTime=1
  Logical Operator1 : Logic  Operator=OR  IconShape=distinctive  AllPortsSameDT=off  OutDataTypeStr=boolean
  Logical Operator2 : Logic  Operator=NOT  IconShape=distinctive  AllPortsSameDT=off  OutDataTypeStr=boolean
  Logical Operator3 : Logic  Operator=OR  IconShape=distinctive  AllPortsSameDT=off  OutDataTypeStr=boolean
  State Control : StateControl  StateControl=Synchronous
  Terminator : Terminator
  Unit Delay Enabled Synchronous : hdlsllib/Discrete/Unit Delay Enabled Synchronous  InitialCondition=0.0  SampleTime=-1
  rising_edge_detector : $bdroot/rising_edge_detector  SystemSampleTime=-1  VariantActivationTime=update diagram  AllowFlexibleInterface=on  Latency=0  AutoFrameSizeCalculation=off
  ready : Outport  VectorParamsAs1DForOutWhenUnconnected=off
  wires:
  Delay/1 -> Logical Operator3/1
  new_psdu/1 -> Logical Operator1/2
  rising_edge_detector/1 -> Logical Operator1/1
  Logical Operator1/1 -> Delay/1
  next_frame/1 -> rising_edge_detector/1
  HDL Counter/2 -> Logical Operator2/1, Logical Operator3/2
  Logical Operator3/1 -> Unit Delay Enabled Synchronous/2
  Unit Delay Enabled Synchronous/1 -> ready/1, HDL Counter/1
  HDL Counter/1 -> Terminator/1
  Logical Operator2/1 -> Unit Delay Enabled Synchronous/1

== system HDL_ieee_8021513/full_rx/LDPC_shared ==
  ldpc_data_header : Inport
  ldpc_ctrl_header : Inport  Port=2
  ldpc_data_payload : Inport  Port=3
  ldpc_ctrl_payload : Inport  Port=4
  start_header : Inport  Port=5
  end_header : Inport  Port=6
  Constant{,1..5} (6 alike) : Constant  Value=0  OutDataTypeStr=boolean  SampleTime=-1
  Delay{,1..8} (9 alike) : Delay  DelayLength=1  InitialCondition=0  UseCircularBuffer=on
  LDPC Decoder : whdledac/LDPC Decoder  ParityCheckMatrix=CONST.Hc_12H  BlockSize=14  Algorithm=Min-sum  ScalingFactor=0.75  Termination=Max  SpecifyInputs=Property  NumIterations=CONST.ldpcDecoderMaxNumberIterations  MaxNumIterations=8  ParityCheckStatus=off  SimulateUsing=Code generation
  OR : Logic  Operator=OR  IconShape=distinctive  AllPortsSameDT=off  OutDataTypeStr=boolean
  Sample Control Bus Creator : whdlutilities/Sample Control Bus Creator
  Sample Control Bus Creator1 : whdlutilities/Sample Control Bus Creator
  Sample Control Bus Creator2 : whdlutilities/Sample Control Bus Creator
  Sample Control Bus Selector : whdlutilities/Sample Control Bus Selector  OutputSignals=start,end,valid
  Sample Control Bus Selector1 : whdlutilities/Sample Control Bus Selector  OutputSignals=start,end,valid
  Sample Control Bus Selector2 : whdlutilities/Sample Control Bus Selector  OutputSignals=start,end,valid
  Switch{,2..10} (10 alike) : Switch  Criteria=u2 ~= 0  SaturateOnIntegerOverflow=off  InputSameDT=off
  Switch1 : Switch  Criteria=u2 ~= 0  SaturateOnIntegerOverflow=off
  Unit Delay : UnitDelay  SampleTime=-1  HasFrameUpgradeWarning=on
  ldpc_data_out : Outport
  ldpc_ctrl_header_out : Outport  Port=2
  ldpc_ctrl_payload_out : Outport  Port=3
  ldpc_next_frame : Outport  Port=4
  wires:
  Constant3/1 -> Switch10/1
  Constant4/1 -> Switch9/1
  Constant5/1 -> Switch8/1
  Delay3/1 -> ldpc_data_out/1
  Delay2/1 -> ldpc_next_frame/1
  Delay1/1 -> ldpc_ctrl_payload_out/1
  [is_header] -> Switch8/2
  Sample Control Bus Creator2/1 -> Delay1/1
  [is_header] -> Switch10/2
  Switch10/1 -> Sample Control Bus Creator2/3
  Switch8/1 -> Sample Control Bus Creator2/1
  [is_header] -> Switch9/2
  Switch9/1 -> Sample Control Bus Creator2/2
  Delay/1 -> ldpc_ctrl_header_out/1
  Sample Control Bus Creator1/1 -> Delay/1
  Switch7/1 -> Sample Control Bus Creator1/3
  Switch6/1 -> Sample Control Bus Creator1/2
  Switch5/1 -> Sample Control Bus Creator1/1
  Constant2/1 -> Switch5/3
  Constant1/1 -> Switch6/3
  [is_header] -> Switch5/2
  [is_header] -> Switch6/2
  [is_header] -> Switch7/2
  Constant/1 -> Switch7/3
  Sample Control Bus Selector2/3 -> Switch7/1, Switch10/3
  Sample Control Bus Selector2/2 -> Switch6/1, Switch9/3
  Sample Control Bus Selector2/1 -> Switch5/1, Switch8/3
  Delay7/1 -> Sample Control Bus Selector2/1
  [is_header] -> Switch4/2
  [is_header] -> Switch3/2
  [is_header] -> Switch2/2
  [is_header] -> Switch/2
  Sample Control Bus Creator/1 -> Delay5/1
  Switch4/1 -> Sample Control Bus Creator/3
  Sample Control Bus Selector/2 -> Switch3/1
  ldpc_data_payload/1 -> Switch/3
  Sample Control Bus Selector/1 -> Switch2/1
  Delay4/1 -> LDPC Decoder/1
  LDPC Decoder/2 -> Delay7/1
  Switch/1 -> Delay4/1
  Delay6/1 -> Delay3/1
  Delay5/1 -> LDPC Decoder/2
  Switch2/1 -> Sample Control Bus Creator/1
  Unit Delay/1 -> Switch1/3
  ldpc_ctrl_header/1 -> Sample Control Bus Selector/1
  LDPC Decoder/3 -> Delay8/1
  ldpc_ctrl_payload/1 -> Sample Control Bus Selector1/1
  Sample Control Bus Selector1/2 -> Switch3/3
  LDPC Decoder/1 -> Delay6/1
  Switch3/1 -> Sample Control Bus Creator/2
  ldpc_data_header/1 -> Switch/1
  Switch1/1 -> Unit Delay/1, [is_header]
  Sample Control Bus Selector1/3 -> Switch4/3
  start_header/1 -> Switch1/1, OR/1
  OR/1 -> Switch1/2
  end_header/1 -> OR/2
  Sample Control Bus Selector/3 -> Switch4/1
  Delay8/1 -> Delay2/1
  Sample Control Bus Selector1/1 -> Switch2/3

== system HDL_ieee_8021513/full_rx/cpid_to_cplen ==
  cp_id : Inport
  Bits to Word : hdlsllib/Logic and Bit Operations/Bits to Word
  Constant3 : Constant  Value=CONST.N/32  OutDataTypeStr=fixdt(0,4,0)  SampleTime=-1
  Data Type Conversion : DataTypeConversion  OutDataTypeStr=fixdt(0,1,0)  SaturateOnIntegerOverflow=off  RndMeth=Floor
  Delay1 : Delay  DelayLength=1  InitialCondition=0  UseCircularBuffer=on
  Product : Product  OutDataTypeStr=uint8
  payload_cp_len : Outport
  wires:
  cp_id/1 -> Data Type Conversion/1
  Data Type Conversion/1 -> Bits to Word/1
  Product/1 -> Delay1/1
  Bits to Word/1 -> Product/2
  Constant3/1 -> Product/1
  Delay1/1 -> payload_cp_len/1

== system HDL_ieee_8021513/full_rx/header_clock_x2 ==
  data_in : Inport
  valid_header : Inport  Port=2
  Serializer1D : hdlsllib/HDL Operations/Serializer1D  Ratio=2  IdleCycles=0  validIn=on  startOut=off  validOut=on  inputDataDimensions=-1  inputSampleTime=-1  inputSignalType=auto
  rising_edge_detector : $bdroot/rising_edge_detector  SystemSampleTime=-1  VariantActivationTime=update diagram  AllowFlexibleInterface=on  Latency=0  AutoFrameSizeCalculation=off
  data_out : Outport
  start : Outport  Port=2
  wires:
  rising_edge_detector/1 -> start/1
  valid_header/1 -> Serializer1D/2
  Serializer1D/1 -> data_out/1
  Serializer1D/2 -> rising_edge_detector/1
  data_in/1 -> Serializer1D/1

== system HDL_ieee_8021513/full_rx/prepare_payload_data ==
  note: Note_ this counter makes sure that the fifo always has data, and is not emptied in the middle of an LDPC block
  note: Maximum value is 3741
  data_in : Inport
  valid_payload : Inport  Port=2
  payload_ready : Inport  Port=3
  reset : Inport  Port=4
  Delay : Delay  DelayLength=1  InitialCondition=0  UseCircularBuffer=on
  Delay2 : Delay  DelayLength=1  InitialCondition=0  UseCircularBuffer=on
  HDL Counter1 : hdlsllib/Sources/HDL Counter  CountType=Count limited  CountInit=0  CountStep=1  CountMax=CONST.rxDelayBeforeReadingFIFOPayload  CountFromType=Initial value  CountFrom=0  CountResetPort=off  CountLoadPort=off  CountEnbPort=on  CountDirPort=off  CountHitOutputPort=on  CountDataType=Unsigned  CountWordLen=14  CountFracLen=0  CountSampTime=1
  HDL FIFO : hdlsllib/HDL RAMs/HDL FIFO  fifo_size=CONST.FIFORxPayloadSize  mode=Classic  ratio=1  push_msg=Error  pop_msg=Error  show_empty=on  show_full=off  show_num=on  LabelModeActiveChoice_Mode=Classic  rst_port=on
  Logical Operator2 : Logic  IconShape=distinctive  AllPortsSameDT=off  OutDataTypeStr=boolean
  Logical Operator3 : Logic  Operator=NOT  IconShape=distinctive  AllPortsSameDT=off  OutDataTypeStr=boolean
  OR1 : Logic  Operator=OR  IconShape=distinctive  AllPortsSameDT=off  OutDataTypeStr=boolean
  Switch1 : Switch  Criteria=u2 ~= 0  SaturateOnIntegerOverflow=off  InputSameDT=off
  Terminator : Terminator
  Terminator1 : Terminator
  Unit Delay1 : UnitDelay  SampleTime=-1  HasFrameUpgradeWarning=on
  falling_edge_detector1 : $bdroot/falling_edge_detector  SystemSampleTime=-1  VariantActivationTime=update diagram  AllowFlexibleInterface=on  Latency=0  AutoFrameSizeCalculation=off
  payload_clock_x2 : Subsystem
  dataOut : Outport
  valid_in : Outport  Port=2
  new_frame : Outport  Port=3
  wires:
  reset/1 -> HDL FIFO/4
  HDL FIFO/3 -> Terminator/1  "fifo_payload"
  Delay2/1 -> OR1/2
  HDL Counter1/1 -> Terminator1/1
  OR1/1 -> Switch1/2
  falling_edge_detector1/1 -> OR1/1, Switch1/1
  HDL Counter1/2 -> Delay2/1, new_frame/1  "new_frame"
  Unit Delay1/1 -> Switch1/3
  Switch1/1 -> HDL Counter1/1, Unit Delay1/1
  HDL FIFO/2 -> Logical Operator3/1, falling_edge_detector1/1  "fifo_empty"
  data_in/1 -> payload_clock_x2/1(data_in)
  payload_clock_x2/2(valid_out) -> HDL FIFO/2  "push"
  payload_clock_x2/1(data_out) -> HDL FIFO/1  "dataIn"
  HDL FIFO/1 -> dataOut/1  "dataOut"
  valid_payload/1 -> payload_clock_x2/2(valid_in)
  Logical Operator2/1 -> HDL FIFO/3, Delay/1
  Delay/1 -> valid_in/1  "valid_in"
  Logical Operator3/1 -> Logical Operator2/1
  payload_ready/1 -> Logical Operator2/2  "payload_ready"

== system HDL_ieee_8021513/full_rx/signal_ack ==
  signal_in : Inport
  free_signal : Inport  Port=2
  Logical Operator : Logic  Operator=OR  IconShape=distinctive  AllPortsSameDT=off  OutDataTypeStr=boolean
  Switch : Switch  Criteria=u2 ~= 0  SaturateOnIntegerOverflow=off  InputSameDT=off
  Unit Delay : UnitDelay  SampleTime=-1  HasFrameUpgradeWarning=on
  rising_edge_detector : $bdroot/rising_edge_detector  SystemSampleTime=-1  VariantActivationTime=update diagram  AllowFlexibleInterface=on  Latency=0  AutoFrameSizeCalculation=off
  signal_out : Outport
  wires:
  free_signal/1 -> Logical Operator/2
  rising_edge_detector/1 -> Switch/1, Logical Operator/1
  Unit Delay/1 -> Switch/3
  Logical Operator/1 -> Switch/2
  Switch/1 -> signal_out/1, Unit Delay/1
  signal_in/1 -> rising_edge_detector/1

== system HDL_ieee_8021513/full_tx/clock_crossing ==
  preamble_in : Inport
  preamble_ctrl_in : Inport  Port=2
  channel : Inport  Port=3
  channel_ctrl : Inport  Port=4
  header_in : Inport  Port=5
  header_ctrl_in : Inport  Port=6
  payload_in : Inport  Port=7
  payload_ctrl_in : Inport  Port=8
  cp_len_in : Inport  Port=9
  payload_len_in : Inport  Port=10
  bits_per_subcarrier_in : Inport  Port=11
  Deserializer1D : hdlsllib/HDL Operations/Deserializer1D  Ratio=2  IdleCycles=0  InitialCondition=0  startIn=off  validIn=on  validOut=on  inputDataDimensions=-1  inputSampleTime=-1  inputSignalType=auto
  Deserializer1D1 : hdlsllib/HDL Operations/Deserializer1D  Ratio=2  IdleCycles=0  InitialCondition=0  startIn=off  validIn=on  validOut=on  inputDataDimensions=-1  inputSampleTime=-1  inputSignalType=auto
  Rate Transition : RateTransition  OutPortSampleTime=1/CONST.fPHY
  Rate Transition1 : RateTransition  OutPortSampleTime=1/CONST.fPHY
  Rate Transition2 : RateTransition  OutPortSampleTime=1/CONST.fPHY
  Sample Control Bus Selector{,1..3} (4 alike) : whdlutilities/Sample Control Bus Selector  OutputSignals=start,end,valid
  State Control : StateControl  StateControl=Synchronous
  Terminator{,1..7} (8 alike) : Terminator
  preamble_out : Outport
  preamble_valid : Outport  Port=2
  channel_out : Outport  Port=3
  channel_valid : Outport  Port=4
  header_out : Outport  Port=5
  header_valid : Outport  Port=6
  payload_out : Outport  Port=7
  payload_valid_out : Outport  Port=8
  payload_len_out : Outport  Port=9  VectorParamsAs1DForOutWhenUnconnected=off
  bits_per_subcarrier_out : Outport  Port=10  VectorParamsAs1DForOutWhenUnconnected=off
  cp_len_out : Outport  Port=11  VectorParamsAs1DForOutWhenUnconnected=off
  wires:
  preamble_ctrl_in/1 -> Sample Control Bus Selector/1
  Sample Control Bus Selector/1 -> Terminator/1  "<start>"
  Sample Control Bus Selector/2 -> Terminator1/1  "<end>"
  Sample Control Bus Selector/3 -> preamble_valid/1  "<valid>"
  preamble_in/1 -> preamble_out/1
  Sample Control Bus Selector1/3 -> channel_valid/1  "<valid>"
  channel_ctrl/1 -> Sample Control Bus Selector1/1
  Sample Control Bus Selector1/2 -> Terminator3/1  "<end>"
  Sample Control Bus Selector1/1 -> Terminator2/1  "<start>"
  channel/1 -> channel_out/1
  Sample Control Bus Selector2/1 -> Terminator5/1  "<start>"
  Deserializer1D/1 -> header_out/1
  Sample Control Bus Selector2/2 -> Terminator4/1  "<end>"
  Deserializer1D/2 -> header_valid/1
  header_ctrl_in/1 -> Sample Control Bus Selector2/1
  Sample Control Bus Selector2/3 -> Deserializer1D/2  "<valid>"
  header_in/1 -> Deserializer1D/1
  Sample Control Bus Selector3/1 -> Terminator7/1  "<start>"
  Deserializer1D1/2 -> payload_valid_out/1
  Sample Control Bus Selector3/2 -> Terminator6/1  "<end>"
  payload_ctrl_in/1 -> Sample Control Bus Selector3/1
  Deserializer1D1/1 -> payload_out/1
  Sample Control Bus Selector3/3 -> Deserializer1D1/2  "<valid>"
  payload_in/1 -> Deserializer1D1/1
  bits_per_subcarrier_in/1 -> Rate Transition2/1
  payload_len_in/1 -> Rate Transition1/1
  cp_len_in/1 -> Rate Transition/1
  Rate Transition/1 -> cp_len_out/1
  Rate Transition1/1 -> payload_len_out/1
  Rate Transition2/1 -> bits_per_subcarrier_out/1
